simulink model "FBL"  (R2021a)
settings: Solver=VariableStepAuto  StartTime=0.0  StopTime=10.0  RelTol=1e-3
undefined symbols (not defined in the file): Levenberg, Marquardt
libraries: robotmaniplib x12, robotcorelib x3, pid_lib x1
settings Model: Creator=ASUS  LastModifiedBy=ASUS

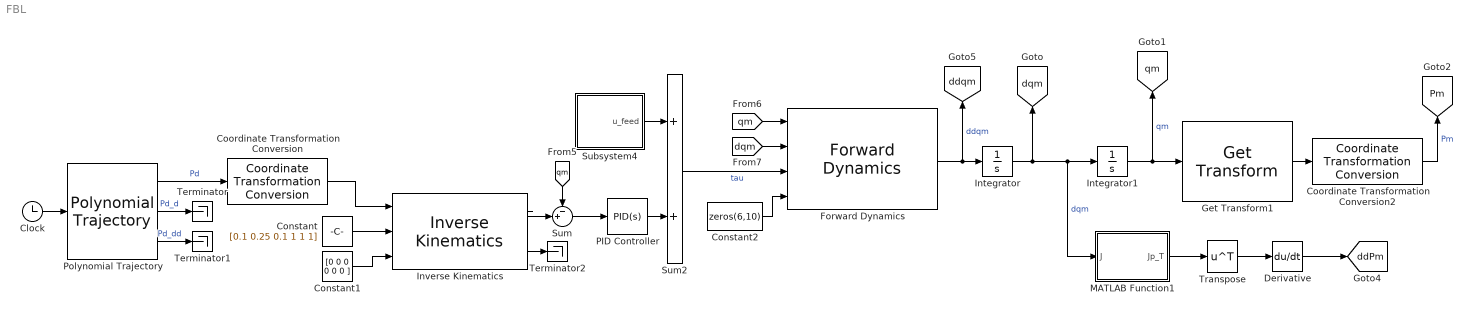
== system FBL ==
  Clock : Clock
  Constant : Constant  Value=[0.1 0.25 0.1 1 1 1]
  Constant1 : Constant  Value=[0 0 0 0 0 0 ]
  Constant2 : Constant  Value=zeros(6,10)
  Coordinate Transformation Conversion : robotcorelib/Coordinate Transformation Conversion  InputRepresentation=Translation Vector  InputEulerSequence=ZYX  ShowTrVecInputPort=on  OutputRepresentation=Homogeneous Transformation  OutputEulerSequence=ZYX  ShowTrVecOutputPort=on  SimulateUsing=Interpreted execution
      settings: SourceProductBaseCode=NV,RO,RR,UV
  Coordinate Transformation Conversion2 : robotcorelib/Coordinate Transformation Conversion  InputRepresentation=Homogeneous Transformation  InputEulerSequence=ZYX  ShowTrVecInputPort=on  OutputRepresentation=Translation Vector  OutputEulerSequence=ZYX  ShowTrVecOutputPort=on  SimulateUsing=Code generation
      settings: SourceProductBaseCode=NV,RO,RR,UV
  Derivative : Derivative
  Forward Dynamics : robotmaniplib/Forward Dynamics  RigidBodyTree=robot  SimulateUsing=Code generation
  Get Transform1 : robotmaniplib/Get Transform  RigidBodyTree=robot  SourceBody=tool0  TargetBody=world  SimulateUsing=Code generation
  Integrator : Integrator  InitialCondition=0.01
  Integrator1 : Integrator  InitialCondition=0.01
  Inverse Kinematics : robotmaniplib/Inverse Kinematics  RigidBodyTree=robot  EndEffector=tool0  ShowInfo=on  SolverName=Levenberg-Marquardt  EnforceJointLimits=on  MaxIterations=1500  MaxTime=10  GradientTolerance=1e-3  SolutionTolerance=1e-3  StepTolerance=1e-14  ErrorChangeTolerance=1e-12  UseErrorDamping=on  DampingBias=0.0025  SimulateUsing=Interpreted execution
  MATLAB Function1 : MATLAB Function  TreatAsAtomicUnit=on
  PID Controller : pid_lib/PID Controller  Controller=PID  Form=Parallel  TimeDomain=Continuous-time  UseExternalTs=off  SampleTime=-1  IntegratorMethod=Forward Euler  FilterMethod=Forward Euler  ControllerParametersSource=internal  P=1  I=1  D=0  UseFilter=on  N=100  TunerSelectOption=Transfer Function Based (PID Tuner App)  InitialConditionSource=internal  InitialConditionForIntegrator=0  InitialConditionForFilter=0  DifferentiatorICPrevScaledInput=0  ExternalReset=none  TrackingMode=off  Kt=1  LimitOutput=off  SatLimitsSource=internal  UpperSaturationLimit=inf  LowerSaturationLimit=-inf  LinearizeAsGain=on  AntiWindupMode=none  Kb=1  POutMin=[]  POutMax=[]  IOutMin=[]  IOutMax=[]  DOutMin=[]  DOutMax=[]  NOutMin=[]  NOutMax=[]  SumOutMin=[]  SumOutMax=[]  SaturationOutMin=[]  SaturationOutMax=[]  PParamMin=[]  PParamMax=[]  IParamMin=[]  IParamMax=[]  DParamMin=[]  DParamMax=[]  NParamMin=[]  NParamMax=[]  KbParamMin=[]  KbParamMax=[]  KtParamMin=[]  KtParamMax=[]  KbOutMin=[]  KbOutMax=[]  KtOutMin=[]  KtOutMax=[]  IntegratorOutMin=[]  IntegratorOutMax=[]  FilterOutMin=[]  FilterOutMax=[]  SumI1OutMin=[]  SumI1OutMax=[]  SumI2OutMin=[]  SumI2OutMax=[]  SumI3OutMin=[]  SumI3OutMax=[]  SumI4OutMin=[]  SumI4OutMax=[]  SumDOutMin=[]  SumDOutMax=[]  DifferentiatorOutMin=[]  DifferentiatorOutMax=[]  FilterDiffOutCoefMin=[]  FilterDiffOutCoefMax=[]  ReciprocalOutMin=[]  ReciprocalOutMax=[]  SumDenOutMin=[]  SumDenOutMax=[]  SumNumOutMin=[]  SumNumOutMax=[]  DivideOutMin=[]  DivideOutMax=[]  UdiffTsProdOutMin=[]  UdiffTsProdOutMax=[]  NTsProdOutMin=[]  NTsProdOutMax=[]  UintegralTsProdOutMin=[]  UintegralTsProdOutMax=[]  UngainTsProdOutMin=[]  UngainTsProdOutMax=[]  IntegratorContinuousStateAttributes=''  IntegratorStateMustResolveToSignalObject=off  IntegratorRTWStateStorageClass=Auto  FilterContinuousStateAttributes=''  FilterStateMustResolveToSignalObject=off  FilterRTWStateStorageClass=Auto  ParallelPVariant=InternalParameters  IdealPVariant=Disabled  IVariant=InternalParameters  DVariant=InternalParameters  IntegratorVariant=Continuous  SatVariant=Disabled  AWVariant=Passthrough  PCopyVariant=Disabled  TRVariant=Disabled  FdbkBlocksVariant=Forward  IdealPFdbkVariant=Disabled  SatFdbkVariant=Disabled  DerivativeFilterVariant=ContFilter  NVariant=InternalParameters  NCopyVariant=Disabled  FilterICVariant=InternalICsFilter  IntegratorICVariant=InternalICs  ExternalResetVariant=Disabled  TRSumVariant=Passthrough  SumFdbkVariant=Disabled  SumVariant=Sum_PID  TsampFilterVariant=InternalTs  TsampNgainVariant=Passthrough  TsampIntegralVariant=Passthrough  ExternalSaturationOutDataTypeStr=Inherit: Same as second input
  Polynomial Trajectory : robotcorelib/Polynomial Trajectory  WaypointSource=Internal  Waypoints=[ 0.1 0.1; 0.2 0.2; 0.3 0.3]  TimePoints=[ 0, 0.01 ]  TimeInterval=[ 1, 4 ]  Method=Cubic Polynomial  ParameterSource=Internal  VelocityBoundaryCondition=zeros( 3, 2 )  AccelerationBoundaryCondition=zeros( 2, 5 )  SimulateUsing=Interpreted execution
  Subsystem4 : Subsystem
  Sum : Sum  Inputs=-+|
  Sum2 : Sum
  Terminator : Terminator
  Terminator1 : Terminator
  Terminator2 : Terminator
  Transpose : Math  Operator=transpose  SaturateOnIntegerOverflow=on
  tag scope: Pm=global, ddPm=global, ddqm=global, dqm=global, qm=global
  wires:
  Clock/1 -> Polynomial Trajectory/1
  Get Transform1/1 -> Coordinate Transformation Conversion2/1
  Forward Dynamics/1 -> Integrator/1, [ddqm]  "ddqm"
  Polynomial Trajectory/3 -> Terminator1/1  "Pd_dd"
  Constant2/1 -> Forward Dynamics/4
  [dqm] -> Forward Dynamics/2
  Polynomial Trajectory/1 -> Coordinate Transformation Conversion/1  "Pd"
  Sum2/1 -> Forward Dynamics/3  "tau"
  [qm] -> Sum/1
  Sum/1 -> PID Controller/1
  Polynomial Trajectory/2 -> Terminator/1  "Pd_d"
  [qm] -> Forward Dynamics/1
  Integrator1/1 -> [qm], Get Transform1/1  "qm"
  Integrator/1 -> MATLAB Function1/1(J), Integrator1/1, [dqm]  "dqm"
  Coordinate Transformation Conversion2/1 -> [Pm]  "Pm"
  MATLAB Function1/1(Jp_T) -> Transpose/1
  Transpose/1 -> Derivative/1
  Derivative/1 -> [ddPm]
  Subsystem4/1(u_feed) -> Sum2/1
  PID Controller/1 -> Sum2/2
  Inverse Kinematics/1 -> Sum/2
  Constant/1 -> Inverse Kinematics/2
  Constant1/1 -> Inverse Kinematics/3
  Coordinate Transformation Conversion/1 -> Inverse Kinematics/1
  Inverse Kinematics/2 -> Terminator2/1

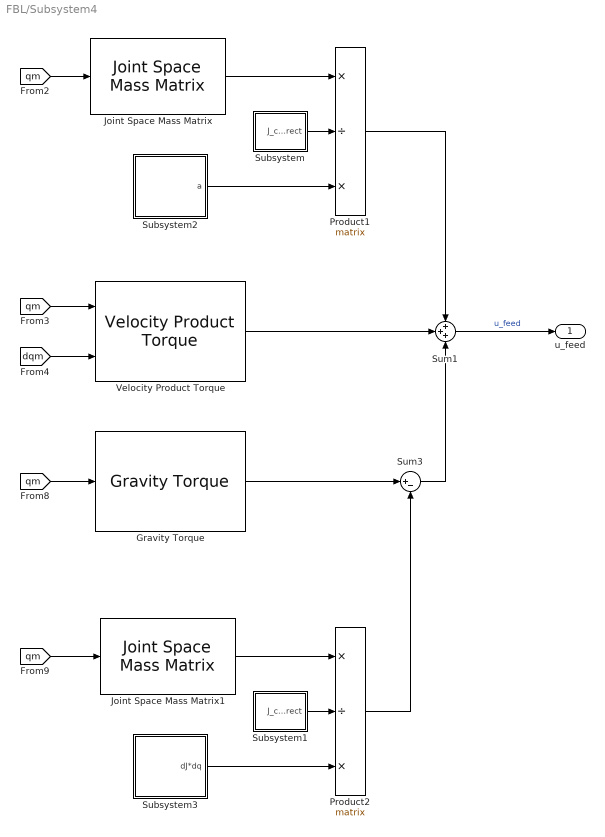
== system FBL/Subsystem4 ==
  Gravity Torque : robotmaniplib/Gravity Torque  RigidBodyTree=robot  SimulateUsing=Interpreted execution
  Joint Space Mass Matrix : robotmaniplib/Joint Space Mass Matrix  RigidBodyTree=robot  SimulateUsing=Interpreted execution
  Joint Space Mass Matrix1 : robotmaniplib/Joint Space Mass Matrix  RigidBodyTree=robot  SimulateUsing=Interpreted execution
  Product1 : Product  Inputs=*/*  Multiplication=Matrix(*)
  Product2 : Product  Inputs=*/*  Multiplication=Matrix(*)
  Subsystem : Subsystem
  Subsystem1 : Subsystem
  Subsystem2 : Subsystem
  Subsystem3 : Subsystem
  Sum1 : Sum  Inputs=+++
  Sum3 : Sum  Inputs=|+-
  Velocity Product Torque : robotmaniplib/Velocity Product Torque  RigidBodyTree=robot  SimulateUsing=Interpreted execution
      settings: SourceProductBaseCode=RO
  u_feed : Outport
  wires:
  [dqm] -> Velocity Product Torque/2
  Subsystem/1(J_correct) -> Product1/2
  Product1/1 -> Sum1/1
  Joint Space Mass Matrix/1 -> Product1/1
  [qm] -> Gravity Torque/1
  [qm] -> Joint Space Mass Matrix/1
  [qm] -> Joint Space Mass Matrix1/1
  Product2/1 -> Sum3/2
  Subsystem3/1(dJ*dq) -> Product2/3
  Velocity Product Torque/1 -> Sum1/2
  Subsystem1/1(J_correct) -> Product2/2
  Joint Space Mass Matrix1/1 -> Product2/1
  Sum3/1 -> Sum1/3
  [qm] -> Velocity Product Torque/1
  Subsystem2/1(a) -> Product1/3
  Gravity Torque/1 -> Sum3/1
  Sum1/1 -> u_feed/1  "u_feed"

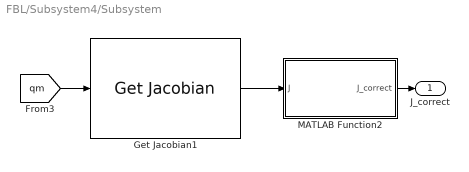
== system FBL/Subsystem4/Subsystem ==
  Get Jacobian1 : robotmaniplib/Get Jacobian  RigidBodyTree=robot  EndEffector=tool0  SimulateUsing=Code generation
      settings: SourceProductBaseCode=RO
  MATLAB Function2 : MATLAB Function  TreatAsAtomicUnit=on
  J_correct : Outport
  wires:
  [qm] -> Get Jacobian1/1
  Get Jacobian1/1 -> MATLAB Function2/1(J)
  MATLAB Function2/1(J_correct) -> J_correct/1

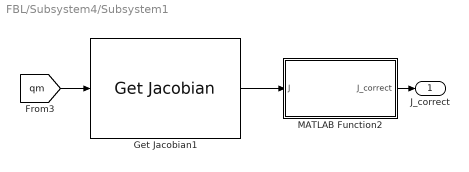
== system FBL/Subsystem4/Subsystem1 ==
  Get Jacobian1 : robotmaniplib/Get Jacobian  RigidBodyTree=robot  EndEffector=tool0  SimulateUsing=Code generation
      settings: SourceProductBaseCode=RO
  MATLAB Function2 : MATLAB Function  TreatAsAtomicUnit=on
  J_correct : Outport
  wires:
  MATLAB Function2/1(J_correct) -> J_correct/1
  Get Jacobian1/1 -> MATLAB Function2/1(J)
  [qm] -> Get Jacobian1/1

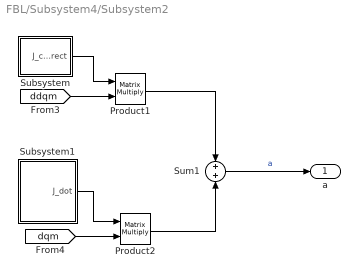
== system FBL/Subsystem4/Subsystem2 ==
  Product1 : Product  Multiplication=Matrix(*)
  Product2 : Product  Multiplication=Matrix(*)
  Subsystem : Subsystem
  Subsystem1 : Subsystem
  Sum1 : Sum  Inputs=+|+
  a : Outport
  wires:
  [dqm] -> Product2/2
  [ddqm] -> Product1/2
  Sum1/1 -> a/1  "a"
  Product2/1 -> Sum1/2
  Subsystem/1(J_correct) -> Product1/1
  Subsystem1/1(J_dot) -> Product2/1
  Product1/1 -> Sum1/1

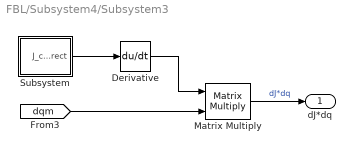
== system FBL/Subsystem4/Subsystem3 ==
  Derivative : Derivative
  Matrix Multiply : Product  Multiplication=Matrix(*)
  Subsystem : Subsystem
  dJ*dq : Outport
  wires:
  Subsystem/1(J_correct) -> Derivative/1
  Matrix Multiply/1 -> dJ*dq/1  "dJ*dq"
  Derivative/1 -> Matrix Multiply/1
  [dqm] -> Matrix Multiply/2

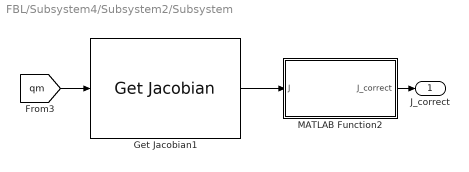
== system FBL/Subsystem4/Subsystem2/Subsystem ==
  Get Jacobian1 : robotmaniplib/Get Jacobian  RigidBodyTree=robot  EndEffector=tool0  SimulateUsing=Code generation
      settings: SourceProductBaseCode=RO
  MATLAB Function2 : MATLAB Function  TreatAsAtomicUnit=on
  J_correct : Outport
  wires:
  [qm] -> Get Jacobian1/1
  Get Jacobian1/1 -> MATLAB Function2/1(J)
  MATLAB Function2/1(J_correct) -> J_correct/1

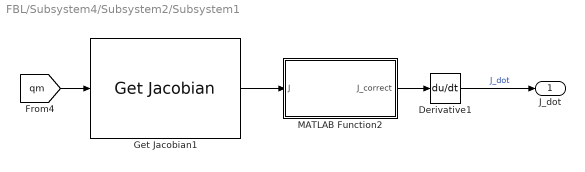
== system FBL/Subsystem4/Subsystem2/Subsystem1 ==
  Derivative1 : Derivative
  Get Jacobian1 : robotmaniplib/Get Jacobian  RigidBodyTree=robot  EndEffector=tool0  SimulateUsing=Code generation
      settings: SourceProductBaseCode=RO
  MATLAB Function2 : MATLAB Function  TreatAsAtomicUnit=on
  J_dot : Outport
  wires:
  [qm] -> Get Jacobian1/1
  MATLAB Function2/1(J_correct) -> Derivative1/1
  Get Jacobian1/1 -> MATLAB Function2/1(J)
  Derivative1/1 -> J_dot/1  "J_dot"

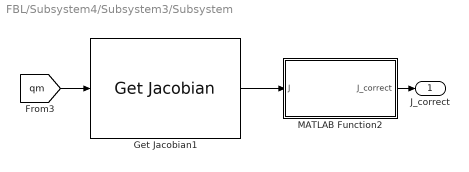
== system FBL/Subsystem4/Subsystem3/Subsystem ==
  Get Jacobian1 : robotmaniplib/Get Jacobian  RigidBodyTree=robot  EndEffector=tool0  SimulateUsing=Code generation
      settings: SourceProductBaseCode=RO
  MATLAB Function2 : MATLAB Function  TreatAsAtomicUnit=on
  J_correct : Outport
  wires:
  MATLAB Function2/1(J_correct) -> J_correct/1
  Get Jacobian1/1 -> MATLAB Function2/1(J)
  [qm] -> Get Jacobian1/1

== matlab function FBL/Subsystem4/Subsystem2/Subsystem/MATLAB Function2 ==
  data: J input; J_correct output
function J_correct = fcn(J)

J_correct = [J(4:6,:);J(1:3,:)];

end

== matlab function FBL/Subsystem4/Subsystem2/Subsystem1/MATLAB Function2 ==
  data: J input; J_correct output
function J_correct = fcn(J)

J_correct = [J(4:6,:);J(1:3,:)];

end

== matlab function FBL/Subsystem4/Subsystem/MATLAB Function2 ==
  data: J input; J_correct output
function J_correct = fcn(J)

J_correct = [J(4:6,:);J(1:3,:)];

end

== matlab function FBL/Subsystem4/Subsystem1/MATLAB Function2 ==
  data: J input; J_correct output
function J_correct = fcn(J)

J_correct = [J(4:6,:);J(1:3,:)];

end

== matlab function FBL/Subsystem4/Subsystem3/Subsystem/MATLAB Function2 ==
  data: J input; J_correct output
function J_correct = fcn(J)

J_correct = [J(4:6,:);J(1:3,:)];

end

== matlab function FBL/MATLAB Function1 ==
  data: J input; Jp_T output
function Jp_T = fcn(J)

Jp_T = J(4:6,:)';

end
